simulink model "lab1ex4"  (R2024a)
settings: Solver=VariableStepAuto  StartTime=0.0  StopTime=50  MaxStep=0.1  RelTol=1e-3
libraries: dspfdesign x2

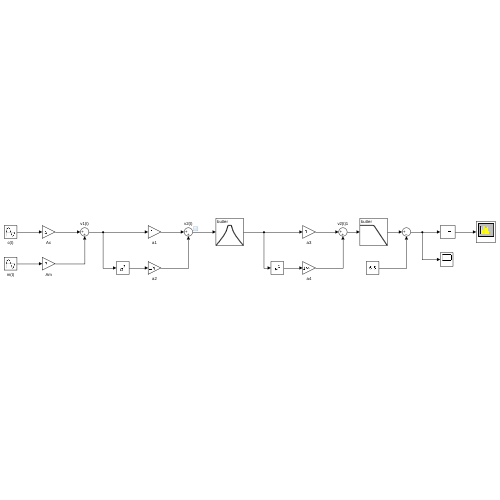
[thumbnail: Simulink's stored preview of the top-level diagram]
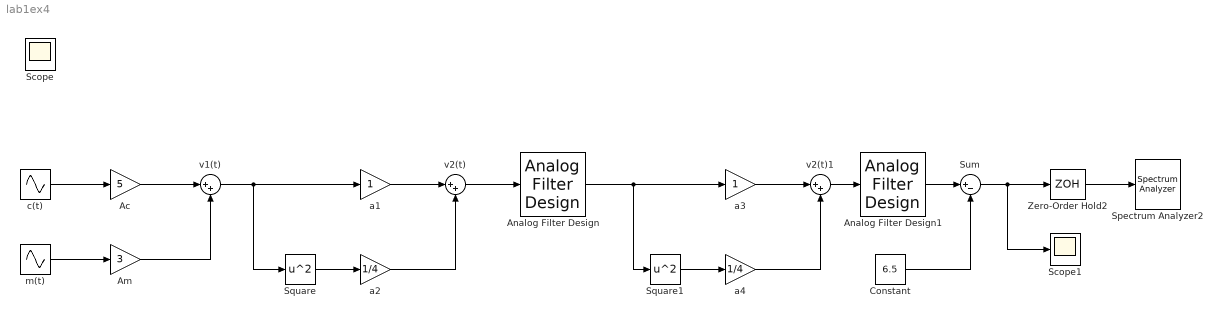
== system lab1ex4 ==
  Ac : Gain  Gain=5
  Am : Gain  Gain=3
  Analog Filter Design : dspfdesign/Analog Filter Design  method=Butterworth  filttype=Bandpass  N=8  Wlo=2*pi*15  Whi=2*pi*25  Rp=2  Rs=40
  Analog Filter Design1 : dspfdesign/Analog Filter Design  method=Butterworth  filttype=Lowpass  N=8  Wlo=2*pi*5  Whi=2*pi*25  Rp=2  Rs=40
  Constant : Constant  Value=6.5
  Scope1 : Scope
  Spectrum Analyzer2 : SpectrumAnalyzer  WindowPosition=[155.000000,45.000000,800.000000,500.000000,]  Visible=on  ScopeFrameLocation=window  PlotAsTwoSidedSpectrum=off  SpectrumUnits=Watts  YLimits=[-4.50776085,40.56984992]
  Square : Math  Operator=square
  Square1 : Math  Operator=square
  Sum : Sum  Inputs=|+-
  Zero-Order Hold2 : ZeroOrderHold  SampleTime=1/100
  a1 : Gain
  a2 : Gain  Gain=1/4
  a3 : Gain
  a4 : Gain  Gain=1/4
  c(t) : Sin  Frequency=2*pi*20  Phase=pi/2  SampleTime=0
  m(t) : Sin  Frequency=2*pi*4  Phase=pi/2  SampleTime=0
  v1(t) : Sum  Inputs=|++
  v2(t) : Sum  Inputs=|++
  v2(t)1 : Sum  Inputs=|++
  Scope : Scope
  wires:
  m(t)/1 -> Am/1
  c(t)/1 -> Ac/1
  Ac/1 -> v1(t)/1
  v1(t)/1 -> a1/1, Square/1
  a1/1 -> v2(t)/1
  a2/1 -> v2(t)/2
  Am/1 -> v1(t)/2
  v2(t)/1 -> Analog Filter Design/1
  Square/1 -> a2/1
  Analog Filter Design/1 -> Square1/1, a3/1
  Square1/1 -> a4/1
  a4/1 -> v2(t)1/2
  v2(t)1/1 -> Analog Filter Design1/1
  a3/1 -> v2(t)1/1
  Zero-Order Hold2/1 -> Spectrum Analyzer2/1
  Analog Filter Design1/1 -> Sum/1
  Constant/1 -> Sum/2
  Sum/1 -> Scope1/1, Zero-Order Hold2/1
